simulink model "sfcndemo_ada_simple_lookup"  (Simulink 6.0)
settings: Solver=FixedStepDiscrete  StartTime=0.0  StopTime=10.0  RelTol=1e-3
PostLoadFcn:
  | tmpStr = get_param(bdroot, 'RTWMakeCommand');incDir = fullfile(matlabroot,'simulink','ada','examples','simple_lookup');tmpStr = strrep(tmpStr, '<INCDIR>', incDir);set_param(bdroot, 'RTWMakeCommand', tmpStr);clear incDir tmpStr;
InitFcn:
  | TableX = linspace(-2, 2, 5)';TableY=exp(-0.5*TableX.*TableX)/sqrt(2*pi);
StopFcn:
  | try,    plot(u,y,'k.', u,yR,'r.', u,yL,'b.');end
CloseFcn:
  | tmpStr = get_param(bdroot, 'RTWMakeCommand');incDir = fullfile(matlabroot,'simulink','ada','examples','simple_lookup');tmpStr = strrep(tmpStr, incDir, '<INCDIR>');set_param(bdroot, 'RTWMakeCommand', tmpStr);clear incDir tmpStr;clear TableX TableY iL iR u y yA yL yR;close;
settings Model: Creator=The MathWorks Inc.  LastModifiedBy=batserve  ExtModeTrigMode=oneshot  ExtModeArmWhenConnect=off  ExtModeAutoUpdateStatusClock=off
settings DataIOCC: LimitDataPoints=off  SaveOutput=off  SaveTime=off  TimeSaveName=t  OutputSaveName=y
settings OptimizationCC: BlockReduction=off  BooleanDataType=off  InlineInvariantSignals=off
settings DebuggingCC: ConsistencyChecking=error  CheckExecutionContextPreStartOutputMsg=on  CheckExecutionContextRuntimeOutputMsg=on  SolverPrmCheckMsg=none
settings HardwareCC: TargetUnknown=on
settings RTWCC: SystemTargetFile=rt_ada_sim.tlc  MakeCommand=make_rtw -ada -ID:\Work\R12\simulink\ada\examples\simple_lookup  TemplateMakefile=gnat_sim.tmf  RetainRTWFile=on  ProcessScript=rt_ada_sim_make_rtw_hook
settings STFCustomTargetCC: TargetFcnLib=ansi_tfl_tmw.mat  GenFloatMathFcnCalls=ANSI_C  ModelReferenceCompliant=off  CombineOutputUpdateFcns=on  MatFileLogging=on  SystemTargetFile=rt_ada_sim.tlc

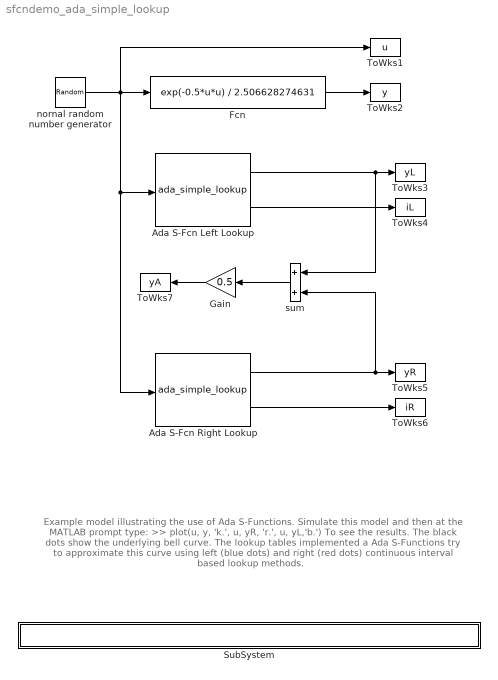
== system sfcndemo_ada_simple_lookup ==
  note: Example model illustrating the use of Ada S-Functions.
      |
      | Simulate this model and then at the MATLAB prompt type:
      |
      | >> plot(u, y, 'k.',  u, yR, 'r.', u, yL,'b.')
      |
      | To see the results. The black dots show the underlying bell curve.
      | The lookup tables implemented a Ada S-Functions try to approximate
      | this curve using left (blue dots) and right (red dots) continuous
      | interval based lookup methods.
  Ada S-Fcn Left Lookup : S-Function  FunctionName=ada_simple_lookup  Parameters=TableX, [TableY;0], 'left'
  Ada S-Fcn Right Lookup : S-Function  FunctionName=ada_simple_lookup  Parameters=TableX, [0;TableY], 'right'
  Fcn : Fcn  Expr=exp(-0.5*u*u) / 2.506628274631
  Gain : Gain  Orientation=left  Gain=0.5  SaturateOnIntegerOverflow=on
  SubSystem : Subsystem  PropExecContextAcrossSSBoundary=on
      settings: OpenFcn=evalin('base','edit(fullfile(matlabroot,''simulink'',''ada'',''examples'',''simple_lookup'',''simple_lookup.adb''))')
      mask Display: disp('matlabroot\simulink\ada\examples\simple_lookup\simple_lookup.adb');
  ToWks1 : ToWorkspace  VariableName=u  SampleTime=-1  SaveFormat=Array
  ToWks2 : ToWorkspace  VariableName=y  SampleTime=-1  SaveFormat=Array
  ToWks3 : ToWorkspace  VariableName=yL  SampleTime=-1  SaveFormat=Array
  ToWks4 : ToWorkspace  VariableName=iL  SampleTime=-1  SaveFormat=Array
  ToWks5 : ToWorkspace  VariableName=yR  SampleTime=-1  SaveFormat=Array
  ToWks6 : ToWorkspace  VariableName=iR  SampleTime=-1  SaveFormat=Array
  ToWks7 : ToWorkspace  VariableName=yA  SampleTime=-1  SaveFormat=Array
  nornal random number generator : RandomNumber  SampleTime=0.01
  sum : Sum  Orientation=left  SaturateOnIntegerOverflow=on  InputSameDT=on
  wires:
  nornal random number generator/1 -> Fcn/1, Ada S-Fcn Left Lookup/1, Ada S-Fcn Right Lookup/1, ToWks1/1
  Fcn/1 -> ToWks2/1
  Ada S-Fcn Left Lookup/2 -> ToWks4/1
  Ada S-Fcn Right Lookup/2 -> ToWks6/1
  Ada S-Fcn Left Lookup/1 -> ToWks3/1, sum/1
  Ada S-Fcn Right Lookup/1 -> ToWks5/1, sum/2
  sum/1 -> Gain/1
  Gain/1 -> ToWks7/1

== system sfcndemo_ada_simple_lookup/SubSystem ==
